simulink model "task_3_schem_1"  (R2024a)
settings: Solver=VariableStepAuto  StartTime=0.0  StopTime=5  RelTol=1e-3
undefined symbols (not defined in the file): A, B, C, D, F_H, G, invCM, M_H, T
settings Model: Creator=user  LastModifiedBy=user

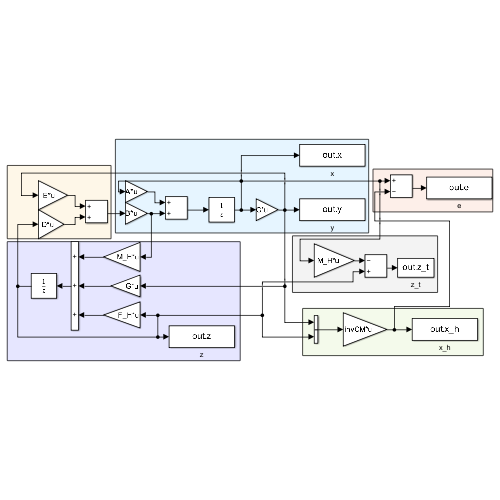
[thumbnail: Simulink's stored preview of the top-level diagram]
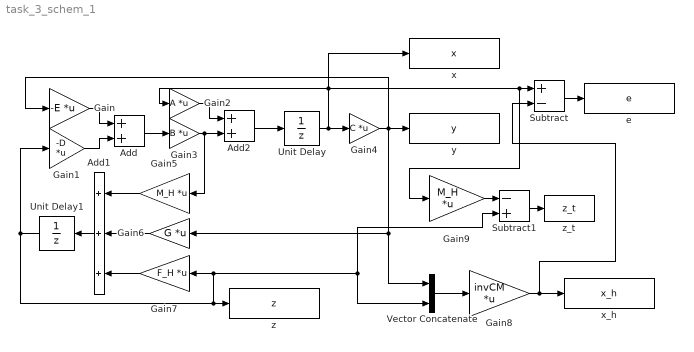
== system task_3_schem_1 ==
  Add : Sum
  Add1 : Sum  Inputs=+++
  Add2 : Sum
  Gain : Gain  Gain=-E  Multiplication=Matrix(K*u)
  Gain1 : Gain  Gain=-D  Multiplication=Matrix(K*u)
  Gain2 : Gain  Gain=A  Multiplication=Matrix(K*u)
  Gain3 : Gain  Gain=B  Multiplication=Matrix(K*u)
  Gain4 : Gain  Gain=C  Multiplication=Matrix(K*u)
  Gain5 : Gain  Gain=M_H  Multiplication=Matrix(K*u)
  Gain6 : Gain  Gain=G  Multiplication=Matrix(K*u)
  Gain7 : Gain  Gain=F_H  Multiplication=Matrix(K*u)
  Gain8 : Gain  Gain=invCM  Multiplication=Matrix(K*u)
  Gain9 : Gain  Gain=M_H  Multiplication=Matrix(K*u)
  Subtract : Sum  Inputs=+-
  Subtract1 : Sum  Inputs=-+
  Unit Delay : UnitDelay  InitialCondition=[1;1]  SampleTime=T  HasFrameUpgradeWarning=on
  Unit Delay1 : UnitDelay  SampleTime=T  HasFrameUpgradeWarning=on
  Vector Concatenate : Concatenate
  e : ToWorkspace  VariableName=e  SaveFormat=Timeseries  SampleTime=-1
  x : ToWorkspace  VariableName=x  SaveFormat=Timeseries  SampleTime=-1
  x_h : ToWorkspace  VariableName=x_h  SaveFormat=Timeseries  SampleTime=-1
  y : ToWorkspace  VariableName=y  SaveFormat=Timeseries  SampleTime=-1
  z : ToWorkspace  VariableName=z  SaveFormat=Timeseries  SampleTime=-1
  z_t : ToWorkspace  VariableName=z_t  SaveFormat=Timeseries  SampleTime=-1
  wires:
  Gain1/1 -> Add/2
  Gain/1 -> Add/1
  Add/1 -> Gain3/1
  Gain3/1 -> Add2/2, Gain5/1
  Gain2/1 -> Add2/1
  Add2/1 -> Unit Delay/1
  Unit Delay/1 -> x/1, Gain2/1, Gain9/1, Subtract/1, Gain4/1
  Gain4/1 -> Vector Concatenate/1, Gain6/1, Gain/1, y/1
  Gain5/1 -> Add1/1
  Gain6/1 -> Add1/2
  Gain7/1 -> Add1/3
  Add1/1 -> Unit Delay1/1
  Unit Delay1/1 -> Subtract1/2, Vector Concatenate/2, Gain7/1, z/1, Gain1/1
  Vector Concatenate/1 -> Gain8/1
  Gain8/1 -> x_h/1, Subtract/2
  Subtract/1 -> e/1
  Subtract1/1 -> z_t/1
  Gain9/1 -> Subtract1/1
